simulink model "btdonghocbai7"  (R2022b)
settings: Solver=VariableStepAuto  StartTime=0.0  StopTime=10.0  RelTol=1e-3
settings Model: Creator=admin  LastModifiedBy=admin

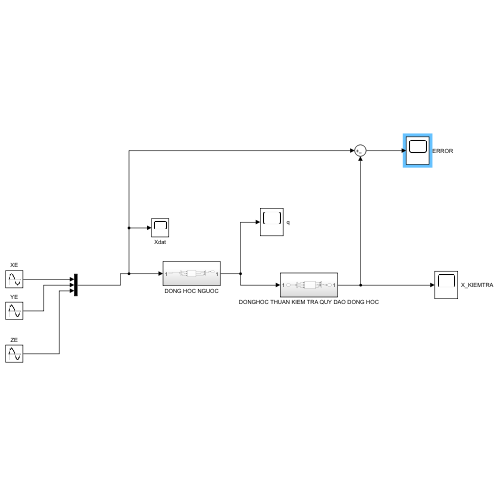
[thumbnail: Simulink's stored preview of the top-level diagram]
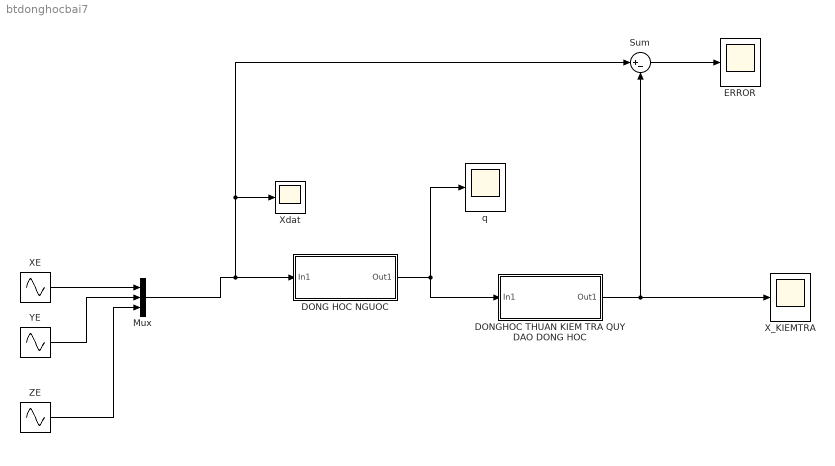
== system btdonghocbai7 ==
  DONG HOC NGUOC : Subsystem
  DONGHOC THUAN KIEM TRA QUY DAO DONG HOC : Subsystem
  ERROR : Scope
  Mux : Mux  Inputs=3
  Sum : Sum  Inputs=|+-
  XE : Sin  Bias=2  Phase=pi  SampleTime=0
  X_KIEMTRA : Scope
  Xdat : Scope
  YE : Sin  Amplitude=1.2  Bias=2  Phase=pi/2  SampleTime=0
  ZE : Sin  Amplitude=1.5  Bias=2  SampleTime=0
  q : Scope
  wires:
  XE/1 -> Mux/1
  YE/1 -> Mux/2
  Mux/1 -> Sum/1, Xdat/1, DONG HOC NGUOC/1(In1)
  DONG HOC NGUOC/1(Out1) -> q/1, DONGHOC THUAN KIEM TRA QUY DAO DONG HOC/1(In1)
  DONGHOC THUAN KIEM TRA QUY DAO DONG HOC/1(Out1) -> X_KIEMTRA/1, Sum/2
  Sum/1 -> ERROR/1
  ZE/1 -> Mux/3

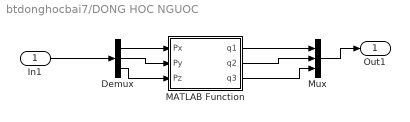
== system btdonghocbai7/DONG HOC NGUOC ==
  In1 : Inport
  Demux : Demux  Outputs=3
  MATLAB Function : MATLAB Function  TreatAsAtomicUnit=on
  Mux : Mux  Inputs=3
  Out1 : Outport
  wires:
  Demux/1 -> MATLAB Function/1(Px)
  Demux/2 -> MATLAB Function/2(Py)
  In1/1 -> Demux/1
  MATLAB Function/1(q1) -> Mux/1
  MATLAB Function/2(q2) -> Mux/2
  Mux/1 -> Out1/1
  Demux/3 -> MATLAB Function/3(Pz)
  MATLAB Function/3(q3) -> Mux/3

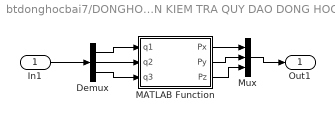
== system btdonghocbai7/DONGHOC THUAN KIEM TRA QUY DAO DONG HOC ==
  In1 : Inport
  Demux : Demux  Outputs=3
  MATLAB Function : MATLAB Function  TreatAsAtomicUnit=on
  Mux : Mux  Inputs=3
  Out1 : Outport
  wires:
  MATLAB Function/1(Px) -> Mux/1
  In1/1 -> Demux/1
  Demux/1 -> MATLAB Function/1(q1)
  Demux/3 -> MATLAB Function/3(q3)
  Demux/2 -> MATLAB Function/2(q2)
  MATLAB Function/2(Py) -> Mux/2
  Mux/1 -> Out1/1
  MATLAB Function/3(Pz) -> Mux/3

== matlab function btdonghocbai7/DONGHOC THUAN KIEM TRA QUY DAO DONG HOC/MATLAB Function ==
  data: Px output; q1 input; Py output; q2 input; q3 input; Pz output
function [Px, Py, Pz] = fcn(q1, q2, q3)
    a2=1;
    a3=1;

    Px=cos(q1)*(a2*cos(q2)+a3*cos(q2 + q3));

    Py=sin(q1)*(a2*cos(q2)+a3*cos(q2 + q3));
    
    Pz=a2*sin(q2)+a3*sin(q2 + q3);
end

== matlab function btdonghocbai7/DONG HOC NGUOC/MATLAB Function ==
  data: Px input; q1 output; Py input; q2 output; Pz input; q3 output
function [q1, q2, q3] = fcn(Px, Py, Pz)
    a2 = 1;
    a3 = 1;

    c3 = (Px^2 + Py^2 + Pz^2 - a2^2 - a3^2)/(2*a2*a3);
    q3 = acos(complex(c3));

    c2 = (sqrt(Px^2+Py^2)*(a2+a3*cos(q3))+Pz*a3*sin(q3))/(a2^2+a3^2+2*a2*a3*cos(q3));
    q2 = acos(complex(c2));


    c1 = Px/(sqrt(Px^2+Py^2));
    q1 = acos(complex(c1));
end
